simulink model "dlbsExamplePeakClassification"  (R2025b)
settings: Solver=FixedStepAuto  StartTime=0.0  StopTime=5e4  FixedStep=1  RelTol=1e-3
undefined symbols (not defined in the file or in its folder): dlbsExamplePeakClassificationStopFcn, out, peaks
libraries: dlbsBlockAdam x6, dlbsBlockDenseLayer x3, simulink x2, dlbsBlockTanh x2, dlbsBlockBceLoss x1, dlbsBlockSigmoid x1
settings Model: Creator=lt6037  LastModifiedBy=lt6037
settings RTWCC: GPUComputeCapability=3.5

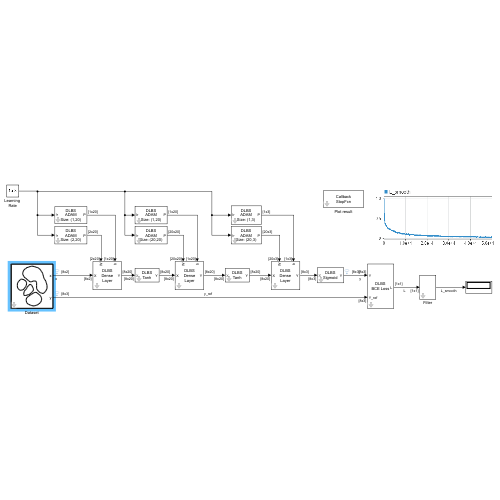
[thumbnail: Simulink's stored preview of the top-level diagram]
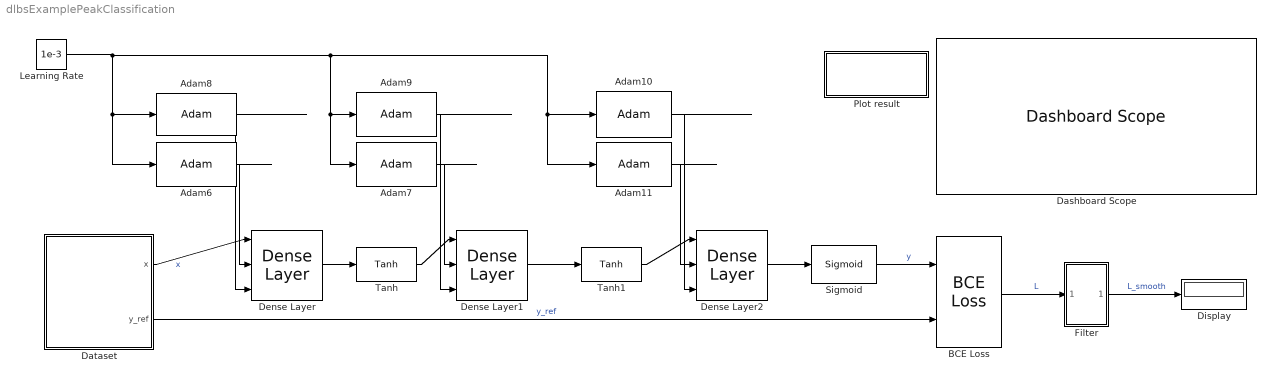
== system dlbsExamplePeakClassification ==
  Adam10 : dlbsBlockAdam/Adam  init=randn(1,3)  beta1=0.9  beta2=0.999  epsilon=1e-8
  Adam11 : dlbsBlockAdam/Adam  init=randn(20,3)  beta1=0.9  beta2=0.999  epsilon=1e-8
  Adam6 : dlbsBlockAdam/Adam  init=randn(2,20)  beta1=0.9  beta2=0.999  epsilon=1e-8
  Adam7 : dlbsBlockAdam/Adam  init=randn(20,20)  beta1=0.9  beta2=0.999  epsilon=1e-8
  Adam8 : dlbsBlockAdam/Adam  init=randn(1,20)  beta1=0.9  beta2=0.999  epsilon=1e-8
  Adam9 : dlbsBlockAdam/Adam  init=randn(1,20)  beta1=0.9  beta2=0.999  epsilon=1e-8
  BCE Loss : dlbsBlockBceLoss/BCE Loss
  Dashboard Scope : DashboardScope  Ymin=0  Ymax=1  FontColor=[0.0, 0.0, 0.0]
  Dataset : Subsystem
      mask Display:
      | [~,~,z] = peaks(30);
      | c = contourc(linspace(-3,3,30),linspace(-3,3,30),z,[-1,1]);
      | 
      | lines = struct.empty();
      | 
      | while ~isempty(c)
      |     l = c(2,1);
      | 
      |     lines(end+1).level = c(1,1);
      |     lines(end).x = c(1,2:l+1);
      |     lines(end).y = c(2,2:l+1);
      |     c(:,1:l+1)=[];
      | end
      | 
      | 
      | for line = lines
      |     plot(line.x,line.y)
      | end
      | 
      | plot(3*[-1,1,1,-1,-1],3*[-1,-1,1,1,-1])
      | 
      | port_label('output', 1, 'x');
      | port_label('output', 2, 'y');
  Dense Layer : dlbsBlockDenseLayer/Dense Layer
  Dense Layer1 : dlbsBlockDenseLayer/Dense Layer
  Dense Layer2 : dlbsBlockDenseLayer/Dense Layer
  Display : Display
  Filter : Subsystem
      mask Display: disp('');
  Learning Rate : Constant  Value=1e-3
  Plot result : Subsystem  StopFcn=dlbsExamplePeakClassificationStopFcn(out);
      mask Display: disp("Callback\nStopFcn")
  Sigmoid : dlbsBlockSigmoid/Sigmoid
  Tanh : dlbsBlockTanh/Tanh
  Tanh1 : dlbsBlockTanh/Tanh
  wires:
  Learning Rate/1 -> Adam10/1, Adam11/1, Adam9/1, Adam7/1, Adam6/1, Adam8/1
  BCE Loss/1 -> Filter/1(In1)  "L"
  Filter/1(loss) -> Display/1  "L_smooth"
  Dataset/2(y_ref) -> BCE Loss/2  "y_ref"
  Sigmoid/1 -> BCE Loss/1  "y"
  Adam6/1 -> Dense Layer/2
  Adam8/1 -> Dense Layer/3
  Adam7/1 -> Dense Layer1/2
  Adam9/1 -> Dense Layer1/3
  Adam10/1 -> Dense Layer2/3
  Adam11/1 -> Dense Layer2/2
  Dense Layer/1 -> Tanh/1
  Dense Layer2/1 -> Sigmoid/1
  Tanh/1 -> Dense Layer1/1
  Dense Layer1/1 -> Tanh1/1
  Tanh1/1 -> Dense Layer2/1
  Dataset/1(x) -> Dense Layer/1  "x"

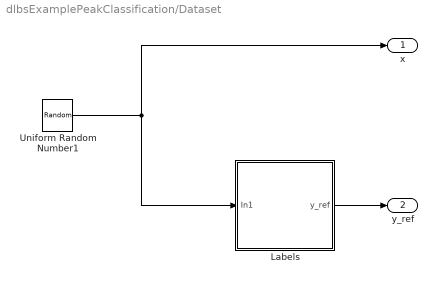
== system dlbsExamplePeakClassification/Dataset ==
  Labels : Subsystem
      mask Display:
      | [~,~,z] = peaks(30);
      | c = contourc(linspace(-3,3,30),linspace(-3,3,30),z,[-1,1]);
      | 
      | lines = struct.empty();
      | 
      | while ~isempty(c)
      |     l = c(2,1);
      | 
      |     lines(end+1).level = c(1,1);
      |     lines(end).x = c(1,2:l+1);
      |     lines(end).y = c(2,2:l+1);
      |     c(:,1:l+1)=[];
      | end
      | 
      | 
      | for line = lines
      |     plot(line.x,line.y)
      | end
      | 
      | plot(3*[-1,1,1,-1,-1],3*[-1,-1,1,1,-1])
  Uniform Random Number1 : UniformRandomNumber  Minimum=-3*ones(8,2)  Maximum=3*ones(8,2)  Seed=randi(2^32,8,2)  SampleTime=1  VectorParams1D=off
  x : Outport
  y_ref : Outport  Port=2
  wires:
  Uniform Random Number1/1 -> x/1, Labels/1(In1)
  Labels/1(y_ref) -> y_ref/1

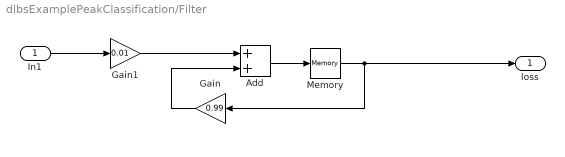
== system dlbsExamplePeakClassification/Filter ==
  In1 : Inport
  Add : Sum
  Gain : Gain  Gain=0.99
  Gain1 : Gain  Gain=0.01
  Memory : Memory  InitialCondition=1
  loss : Outport
  wires:
  Memory/1 -> loss/1, Gain/1
  Gain1/1 -> Add/1
  Gain/1 -> Add/2
  Add/1 -> Memory/1
  In1/1 -> Gain1/1

== system dlbsExamplePeakClassification/Plot result ==

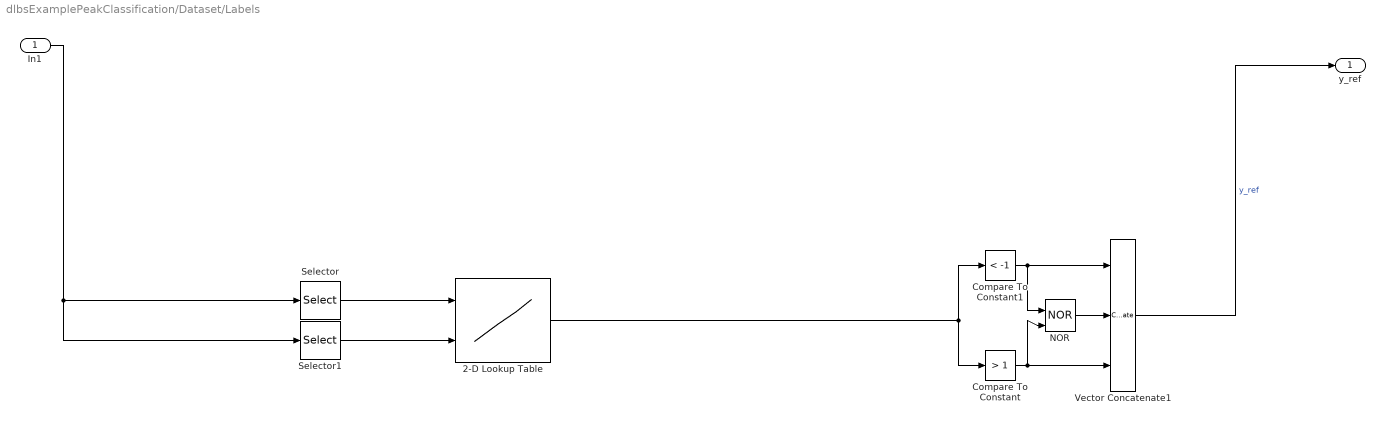
== system dlbsExamplePeakClassification/Dataset/Labels ==
  In1 : Inport
  2-D Lookup Table : Lookup_n-D  BreakpointsForDimension1=linspace(-3,3,30)  BreakpointsForDimension2=linspace(-3,3,30)  Table=peaks(30)  InternalRulePriority=Speed  RndMeth=Simplest
      settings: InputPortMap=u0,u1
  Compare To Constant : simulink/Logic and Bit Operations/Compare To Constant  relop=>  const=1  OutDataTypeStr=boolean
  Compare To Constant1 : simulink/Logic and Bit Operations/Compare To Constant  relop=<  const=-1  OutDataTypeStr=boolean
  NOR : Logic  Operator=NOR  IconShape=distinctive  AllPortsSameDT=off  OutDataTypeStr=boolean
  Selector : Selector  NumberOfDimensions=2  InputPortWidth=3  IndexOptions=Select all,Index vector (dialog)  Indices=[1 3],1  OutputSizes=1,1
  Selector1 : Selector  NumberOfDimensions=2  InputPortWidth=3  IndexOptions=Select all,Index vector (dialog)  Indices=[1 3],2  OutputSizes=1,1
  Vector Concatenate1 : Concatenate  NumInputs=3  Mode=Multidimensional array  ConcatenateDimension=2
  y_ref : Outport
  wires:
  Selector/1 -> 2-D Lookup Table/1
  Compare To Constant1/1 -> Vector Concatenate1/1, NOR/1
  Compare To Constant/1 -> Vector Concatenate1/3, NOR/2
  2-D Lookup Table/1 -> Compare To Constant1/1, Compare To Constant/1
  In1/1 -> Selector/1, Selector1/1
  Selector1/1 -> 2-D Lookup Table/2
  Vector Concatenate1/1 -> y_ref/1  "y_ref"
  NOR/1 -> Vector Concatenate1/2
